simulink model "UAVScenarioModel"  (R2022a)
settings: Solver=VariableStepAuto  StartTime=0.0  StopTime=10.0  RelTol=1e-3
undefined symbols (not defined in the file or in its folder): Lidar, platformUAV
libraries: uavsimlib x6, robotcorelib x1, uavalgslib x1
settings Model: VariantFading=off  Creator=The MathWorks, Inc.  LastModifiedBy=anaveen
settings DebuggingCC: UnconnectedInputMsg=warning  UnconnectedOutputMsg=warning  UnconnectedLineMsg=warning
settings RTWCC: DLArmComputeVersion=19.05

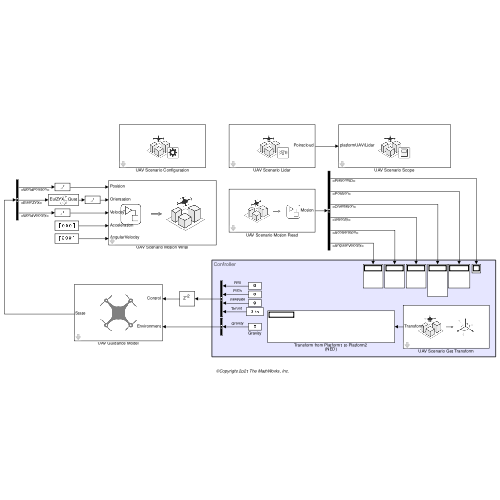
[thumbnail: Simulink's stored preview of the top-level diagram]
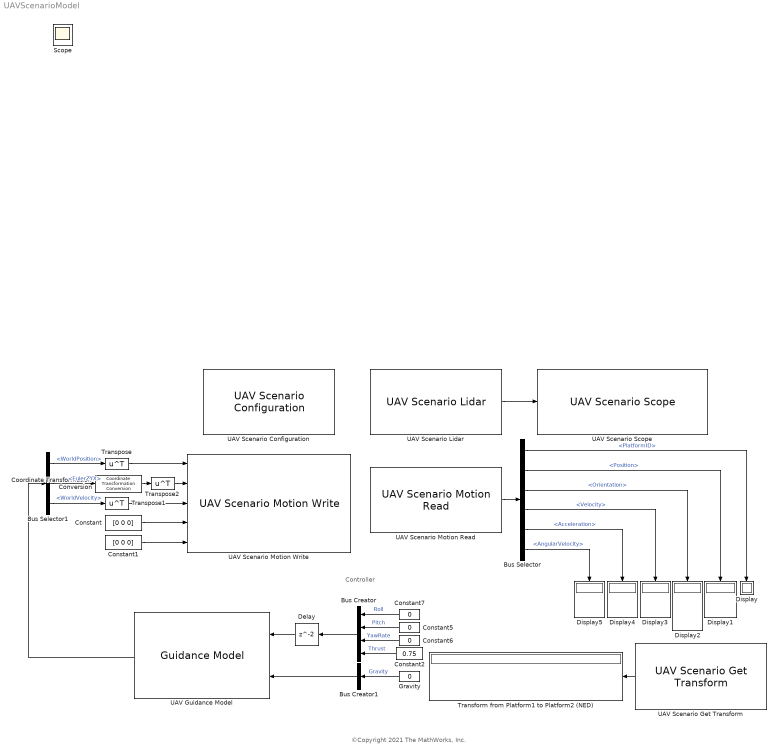
== system UAVScenarioModel ==
  note: ©Copyright 2021 The MathWorks, Inc.
  note: Controller
  Bus Creator : BusCreator  Inputs=4  OutDataTypeStr=Bus: MultirotorGuidanceControlBus  NonVirtualBus=on
  Bus Creator1 : BusCreator  Inputs=1  OutDataTypeStr=Bus: MultirotorGuidanceEnvironmentBus  NonVirtualBus=on
  Bus Selector : BusSelector  OutputSignals=PlatformID,Position,Orientation,Velocity,Acceleration,AngularVelocity
  Bus Selector1 : BusSelector  OutputSignals=WorldPosition,EulerZYX,WorldVelocity
  Constant : Constant  Value=[0 0 0]
  Constant1 : Constant  Value=[0 0 0]
  Constant2 : Constant  Value=0.75
  Constant5 : Constant  Value=0
  Constant6 : Constant  Value=0
  Constant7 : Constant  Value=0
  Coordinate Transformation Conversion : robotcorelib/Coordinate Transformation Conversion  InputRepresentation=Euler Angles  InputEulerSequence=ZYX  ShowTrVecInputPort=on  OutputRepresentation=Quaternion  OutputEulerSequence=ZYX  ShowTrVecOutputPort=on  SimulateUsing=Interpreted execution
      settings: SourceProductBaseCode=RO,NV,RR,UV
  Delay : Delay
  Display{,1..5} (6 alike) : Display
  Gravity : Constant  Value=0
  Transform from Platform1 to Platform2 (NED) : Display
  Transpose : Math  Operator=transpose
  Transpose1 : Math  Operator=transpose
  Transpose2 : Math  Operator=transpose
  UAV Guidance Model : uavalgslib/Guidance Model  ModelType=MultirotorGuidance  SpecifiedDataType=double  SimulateUsing=Interpreted execution  InitialWorldPositionMultirotor=[0; 0; -5]  InitialWorldVelocityMultirotor=[0; 0; 0]  InitialEulerZYXMultirotor=[0; 0; 0]  InitialBodyAngularRateRPYMultirotor=[0; 0; 0]  InitialThrustMultirotor=0  InitialNorthFixedWing=0  InitialEastFixedWing=0  InitialHeightFixedWing=0  InitialAirSpeedFixedWing=0  InitialHeadingAngleFixedWing=0  InitialFlightPathAngleFixedWing=0  InitialRollAngleFixedWing=0  InitialRollAngleRateFixedWing=0  PDRollMultirotor=[3402.97,116.67]  PDPitchMultirotor=[3402.97, 116.67]  PYawRateMultirotor=1950  PThrustMultirotor=3900  MassMultirotor=0.1  PHeightFixedWing=3.9  PHeadingAngleFixedWing=3.9  PFlightPathAngleFixedWing=39  PDRollFixedWing=[3402.97, 116.67]  PAirSpeedFixedWing=1  FlightPathAngleLimitsFixedWing=[-pi/2, pi/2]  StateBusName='MultirotorGuidanceStateBus'  ControlBusName='MultirotorGuidanceControlBus'  EnvironmentBusName='MultirotorGuidanceEnvironmentBus'  DataType=double
      settings: SourceProductBaseCode=UV
  UAV Scenario Configuration : uavsimlib/UAV Scenario Configuration  Priority=-1  UAVScenarioObject=scene  SampleTime=0.1  UpdateParam=false  SensorMotionBusName='SensorMotionBus'  PlatformMotionBusName='PlatformMotionBus'  ScenarioMotionBusName='ScenarioMotionBus'  ScenarioMotionSignalName='ScenarioMotions'
      settings: SourceProductBaseCode=UV
  UAV Scenario Get Transform : uavsimlib/UAV Scenario Get Transform  Priority=1  SourceFrame='platformUAV'  TargetFrame='platformUAV2'
      settings: SourceProductBaseCode=UV
  UAV Scenario Lidar : uavsimlib/UAV Scenario Lidar  Priority=1  SensorName=platformUAV/Lidar  MaxRange=120  RangeAccuracy=0.002  AzimuthLimits=[ -180, 180 ]  AzimuthResolution=0.16  ElevationLimits=[ -20, 20 ]  ElevationResolution=1.25  HasNoise=on  HasOrganizedOutput=on  SampleTime=0.1
      settings: SourceProductBaseCode=UV
  UAV Scenario Motion Read : uavsimlib/UAV Scenario Motion Read  Priority=1  EntityName='platformUAV'  ReferenceFrame=NED
      settings: SourceProductBaseCode=UV
  UAV Scenario Motion Write : uavsimlib/UAV Scenario Motion Write  Priority=0  PlatName='platformUAV'  ReferenceFrame=NED
      settings: SourceProductBaseCode=UV
  UAV Scenario Scope : uavsimlib/UAV Scenario Scope  Priority=1  SensorNameTable={ 'platformUAV/Lidar', 'on' }  SampleTime=0.1
      settings: SourceProductBaseCode=UV
  Scope : Scope
  wires:
  UAV Scenario Lidar/1 -> UAV Scenario Scope/1
  UAV Scenario Motion Read/1 -> Bus Selector/1
  Bus Selector1/1 -> Transpose/1  "<WorldPosition>"
  Bus Selector1/3 -> Transpose1/1  "<WorldVelocity>"
  Bus Selector1/2 -> Coordinate Transformation Conversion/1  "<EulerZYX>"
  Bus Selector/1 -> Display/1  "<PlatformID>"
  Bus Selector/2 -> Display1/1  "<Position>"
  Bus Selector/3 -> Display2/1  "<Orientation>"
  Bus Selector/4 -> Display3/1  "<Velocity>"
  Bus Selector/5 -> Display4/1  "<Acceleration>"
  Bus Selector/6 -> Display5/1  "<AngularVelocity>"
  UAV Scenario Get Transform/1 -> Transform from Platform1 to Platform2 (NED)/1
  Constant/1 -> UAV Scenario Motion Write/4
  Constant1/1 -> UAV Scenario Motion Write/5
  Bus Creator/1 -> Delay/1
  Constant7/1 -> Bus Creator/1  "Roll"
  Constant2/1 -> Bus Creator/4  "Thrust"
  Constant5/1 -> Bus Creator/2  "Pitch"
  Constant6/1 -> Bus Creator/3  "YawRate"
  Gravity/1 -> Bus Creator1/1  "Gravity"
  Transpose1/1 -> UAV Scenario Motion Write/3
  Coordinate Transformation Conversion/1 -> Transpose2/1
  Transpose2/1 -> UAV Scenario Motion Write/2
  Transpose/1 -> UAV Scenario Motion Write/1
  UAV Guidance Model/1 -> Bus Selector1/1
  Delay/1 -> UAV Guidance Model/1
  Bus Creator1/1 -> UAV Guidance Model/2
